simulink model "smokehouse"  (R2022b)
settings: Solver=VariableStepAuto  StartTime=0.0  StopTime=400  RelTol=1e-3
values from neighbouring files (symbols this model uses):
  Ck = 2.34    [constants.m]
  Co = 0.880    (= 0.88)    [constants.m]
  Cu = 0.880    (= 0.88)    [constants.m]
  Cvo = 0.11    [constants.m]
  Cvu = 0.11    [constants.m]
  R1 = 0.625 + 34.61    (= 35.235)    [constants.m]
  R2 = 34.61 + 11.54    (= 46.15)    [constants.m]
  R3 = 34.61 + 115.54    (= 150.15)    [constants.m]
  R4 = 0.625 + 115.54    (= 116.165)    [constants.m]
  R5 = 11.54 + 0.416    (= 11.956)    [constants.m]
  R6 = 0.416 + 115.4    (= 115.816)    [constants.m]
  R7 = 34.61 + 0.29    (= 34.9)    [constants.m]
  R8 = 11.54 + 115.54    (= 127.08)    [constants.m]
libraries: slpidlib x1, simulink x1
settings Model: Creator=juricekm  LastModifiedBy=mluser
settings SolverCC: AlgebraicLoopSolver=TrustRegion
settings DebuggingCC: UnconnectedInputMsg=warning  UnconnectedOutputMsg=warning  UnconnectedLineMsg=warning  SFMachineParentedDataDiag=warning
settings ModelReferenceCC: EnableRefExpFcnMdlSchedulingChecks=on
settings RTWCC: DLArmComputeVersion=19.05

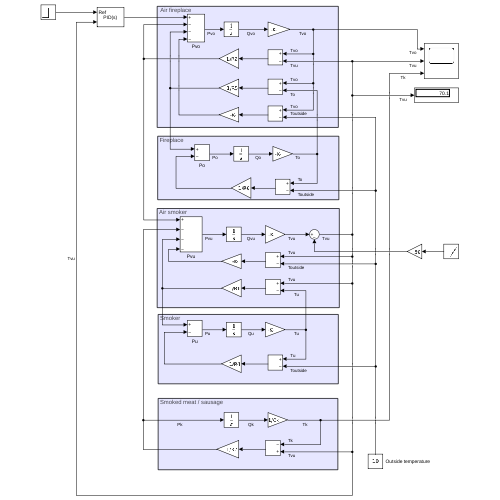
[thumbnail: Simulink's stored preview of the top-level diagram]
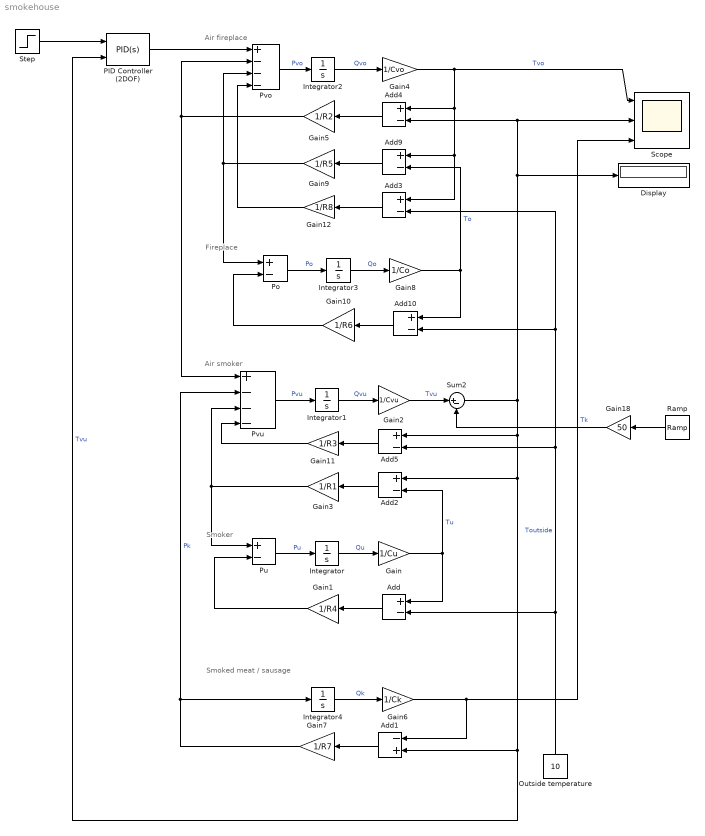
== system smokehouse ==
  note: Fireplace
  note: Air fireplace
  note: Air smoker
  note: Smoker
  note: Smoked meat / sausage
  Add{,2..5,9..10} (7 alike) : Sum  Inputs=+-
  Add1 : Sum  Inputs=-+
  Display : Display
  Gain : Gain  Gain=1/Cu
  Gain1 : Gain  Gain=1/R4
  Gain10 : Gain  Gain=1/R6
  Gain11 : Gain  Gain=1/R3
  Gain12 : Gain  Gain=1/R8
  Gain18 : Gain  Gain=50
  Gain2 : Gain  Gain=1/Cvu
  Gain3 : Gain  Gain=1/R1
  Gain4 : Gain  Gain=1/Cvo
  Gain5 : Gain  Gain=1/R2
  Gain6 : Gain  Gain=1/Ck
  Gain7 : Gain  Gain=1/R7
  Gain8 : Gain  Gain=1/Co
  Gain9 : Gain  Gain=1/R5
  Integrator{,1..4} (5 alike) : Integrator
  Outside temperature : Constant  Value=10
  PID Controller (2DOF) : slpidlib/PID Controller (2DOF)  Controller=PID  Form=Parallel  TimeDomain=Continuous-time  UseExternalTs=off  SampleTime=-1  IntegratorMethod=Forward Euler  FilterMethod=Forward Euler  ControllerParametersSource=internal  P=0.145  I=0.005  UseKiTs=off  D=0.05  N=100  UseFilter=on  b=0.02  c=0.03  TunerSelectOption=Transfer Function Based (PID Tuner App)  InitialConditionSource=internal  InitialConditionForIntegrator=0  InitialConditionForFilter=0  DifferentiatorICPrevScaledInput=0  ExternalReset=none  TrackingMode=off  Kt=1  LimitOutput=off  SatLimitsSource=internal  UpperSaturationLimit=inf  LowerSaturationLimit=-inf  LinearizeAsGain=on  AntiWindupMode=none  Kb=1  LimitIntegrator=off  UpperIntegratorSaturationLimit=inf  LowerIntegratorSaturationLimit=-inf  POutMin=[]  POutMax=[]  IOutMin=[]  IOutMax=[]  DOutMin=[]  DOutMax=[]  NOutMin=[]  NOutMax=[]  bOutMin=[]  bOutMax=[]  cOutMin=[]  cOutMax=[]  SumOutMin=[]  SumOutMax=[]  SaturationOutMin=[]  SaturationOutMax=[]  PParamMin=[]  PParamMax=[]  IParamMin=[]  IParamMax=[]  DParamMin=[]  DParamMax=[]  NParamMin=[]  NParamMax=[]  bParamMin=[]  bParamMax=[]  cParamMin=[]  cParamMax=[]  KbParamMin=[]  KbParamMax=[]  KtParamMin=[]  KtParamMax=[]  KbOutMin=[]  KbOutMax=[]  KtOutMin=[]  KtOutMax=[]  IntegratorOutMin=[]  IntegratorOutMax=[]  FilterOutMin=[]  FilterOutMax=[]  SumI1OutMin=[]  SumI1OutMax=[]  SumI2OutMin=[]  SumI2OutMax=[]  SumI3OutMin=[]  SumI3OutMax=[]  SumI4OutMin=[]  SumI4OutMax=[]  SumDOutMin=[]  SumDOutMax=[]  Sum1OutMin=[]  Sum1OutMax=[]  Sum2OutMin=[]  Sum2OutMax=[]  Sum3OutMin=[]  Sum3OutMax=[]  DifferentiatorOutMin=[]  DifferentiatorOutMax=[]  FilterDiffOutCoefMin=[]  FilterDiffOutCoefMax=[]  ReciprocalOutMin=[]  ReciprocalOutMax=[]  SumDenOutMin=[]  SumDenOutMax=[]  SumNumOutMin=[]  SumNumOutMax=[]  DivideOutMin=[]  DivideOutMax=[]  UdiffTsProdOutMin=[]  UdiffTsProdOutMax=[]  NTsProdOutMin=[]  NTsProdOutMax=[]  UintegralTsProdOutMin=[]  UintegralTsProdOutMax=[]  UngainTsProdOutMin=[]  UngainTsProdOutMax=[]  ClampingZeroOutDataTypeStr=Inherit: Inherit via back propagation  ClampingZeroOutMin=[]  ClampingZeroOutMax=[]  FilterDenConstantOutDataTypeStr=Inherit: Inherit via back propagation  FilterDenConstantOutMin=[]  FilterDenConstantOutMax=[]  PCopyOutDataTypeStr=Inherit: Inherit via back propagation  PCopyOutMin=[]  PCopyOutMax=[]  NCopyOutDataTypeStr=Inherit: Inherit via back propagation  NCopyOutMin=[]  NCopyOutMax=[]  IntegratorContinuousStateAttributes=''  IntegratorStateMustResolveToSignalObject=off  IntegratorRTWStateStorageClass=Auto  FilterContinuousStateAttributes=''  FilterStateMustResolveToSignalObject=off  FilterRTWStateStorageClass=Auto  ParallelPVariant=InternalParameters  IdealPVariant=Disabled  IVariant=InternalParameters  DVariant=InternalParameters  bVariant=InternalParameters  cVariant=InternalParameters  IntegratorVariant=Continuous  SatVariant=Disabled  AWVariant=Passthrough  PCopyVariant=Disabled  TRVariant=Disabled  FdbkBlocksVariant=Forward  IdealPFdbkVariant=Disabled  SatFdbkVariant=Disabled  DerivativeFilterVariant=ContFilter  NVariant=InternalParameters  NCopyVariant=Disabled  FilterICVariant=InternalICsFilter  IntegratorICVariant=InternalICs  ExternalResetVariant=Disabled  TRSumVariant=Passthrough  SumFdbkVariant=Disabled  SumVariant=Sum_PID  TsampFilterVariant=InternalTs  TsampNgainVariant=Passthrough  TsampIntegralVariant=Passthrough  ExternalSaturationOutDataTypeStr=Inherit: Same as second input
  Po : Sum  Inputs=+-
  Pu : Sum  Inputs=+-
  Pvo : Sum  Inputs=+---
  Pvu : Sum  Inputs=+---
  Ramp : simulink/Sources/Ramp  slope=1  start=50  InitialOutput=0
  Scope : Scope  NumInputPorts=3
  Step : Step  After=70  SampleTime=0
  Sum2 : Sum  Inputs=|+-
  wires:
  Integrator/1 -> Gain/1  "Qu"
  Gain/1 -> Add2/2, Add/1  "Tu"
  Pu/1 -> Integrator/1  "Pu"
  Add/1 -> Gain1/1
  Gain1/1 -> Pu/2
  Integrator1/1 -> Gain2/1  "Qvu"
  Sum2/1 -> Add5/1, Add2/1, PID Controller (2DOF)/2, Add1/2, Scope/2, Add4/2, Display/1  "Tvu"
  Add2/1 -> Gain3/1
  Pvu/1 -> Integrator1/1  "Pvu"
  Gain3/1 -> Pvu/3, Pu/1
  Integrator2/1 -> Gain4/1  "Qvo"
  Gain4/1 -> Add9/1, Add3/1, Add4/1, Scope/1  "Tvo"
  Add4/1 -> Gain5/1
  Pvo/1 -> Integrator2/1  "Pvo"
  Outside temperature/1 -> Add3/2, Add10/2, Add5/2, Add/2  "Toutside"
  Integrator3/1 -> Gain8/1  "Qo"
  Add9/1 -> Gain9/1
  Po/1 -> Integrator3/1  "Po"
  Add10/1 -> Gain10/1
  Gain5/1 -> Pvo/2, Pvu/1
  Gain8/1 -> Add9/2, Add10/1  "To"
  Gain9/1 -> Pvo/3, Po/1
  Gain10/1 -> Po/2
  Integrator4/1 -> Gain6/1  "Qk"
  Add1/1 -> Gain7/1
  Gain7/1 -> Integrator4/1, Pvu/2  "Pk"
  Gain6/1 -> Scope/3, Add1/1  "Tk"
  Add5/1 -> Gain11/1
  Gain11/1 -> Pvu/4
  Add3/1 -> Gain12/1
  Gain12/1 -> Pvo/4
  Step/1 -> PID Controller (2DOF)/1
  Gain2/1 -> Sum2/1  "Tvu"
  Ramp/1 -> Gain18/1
  Gain18/1 -> Sum2/2
  PID Controller (2DOF)/1 -> Pvo/1
